simulink model "sim_final_VSS"  (R2019a)
settings: Solver=FixedStepAuto  StartTime=0.0  StopTime=45  FixedStep=1e-2  RelTol=1e-3  EnableMultiTasking=on
values from neighbouring files (symbols this model uses):
  a = 47    [mod1s.m]
  b = -35    [mod1s.m]
  C1 = 0.76    [mod1s.m]
  C2 = 11    [mod1s.m]
  d = 0.5    [mod1s.m]
  ds = 1    [mod1s.m]
  h = 4    [mod1s.m]
  K = 19    [mod1s.m]
  k1 = 3    [mod1s.m]
  k2 = 40    [mod1s.m]
  T = 29    [mod1s.m]
  x0 = -100    [mod1s.m]
  y0 = 0    [mod1s.m]
  z0 = 0    [mod1s.m]
libraries: simulink_extras x1
settings Model: Creator=user  LastModifiedBy=ogure
settings SolverCC: SolverResetMethod=Robust
settings DataIOCC: LimitDataPoints=on  SaveFormat=Array  ReturnWorkspaceOutputs=off  OutputSaveName=x,y,z
settings OptimizationCC: LifeSpan=inf
settings DebuggingCC: SolverPrmCheckMsg=warning  SFUnexpectedBacktrackingDiag=warning  SFNoUnconditionalDefaultTransitionDiag=warning  SFExecutionAtInitializationDiag=none  ArithmeticOperatorsInVariantConditions=warning
settings HardwareCC: ProdBitPerPointer=32  ProdBitPerSizeT=32  ProdBitPerPtrDiffT=32  ProdLargestAtomicFloat=None  ProdIntDivRoundTo=Undefined  ProdEndianess=Unspecified  ProdWordSize=32  ProdHWDeviceType=32-bit Generic
settings ModelReferenceCC: PropagateSignalLabelsOutOfModel=off
settings SFSimCC: SimUseLocalCustomCode=off
settings RTWCC: RTWUseLocalCustomCode=off
settings CodeAppCC: StateflowObjectComments=on
settings GRTTargetCC: TargetLangStandard=C89/C90 (ANSI)  GeneratePreprocessorConditionals=Disable all
settings ConfigComp: CovMetricSettings=dw  CovHtmlReporting=on  CovSaveCumulativeToWorkspaceVar=on  CovSaveSingleToWorkspaceVar=on  CovExternalEMLEnable=off  CovSFcnEnable=off

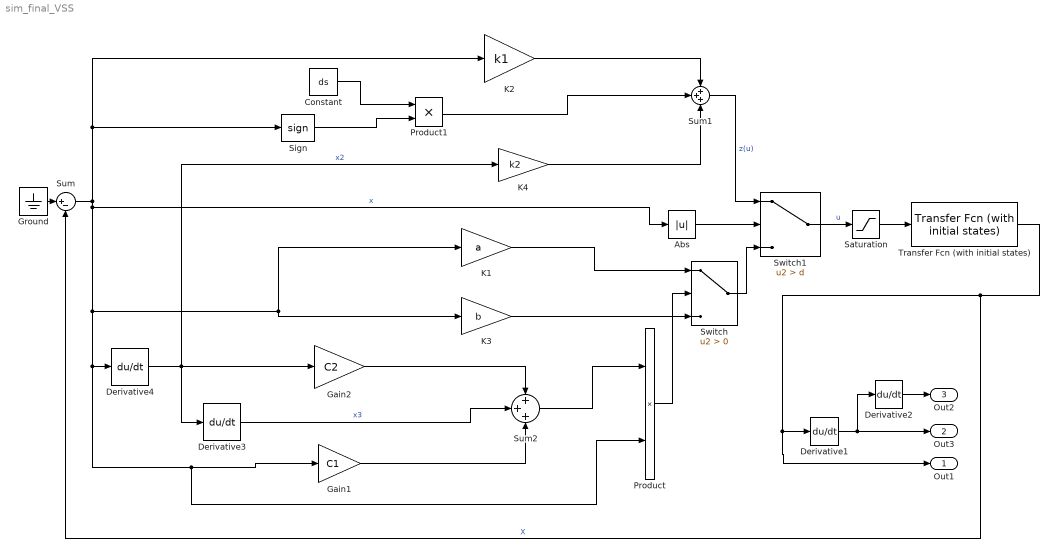
== system sim_final_VSS ==
  Abs : Abs
  Constant : Constant  Value=ds
  Derivative{1..4} (4 alike) : Derivative  CoefficientInTFapproximation=0.00000001
  Gain1 : Gain  Gain=C1
  Gain2 : Gain  Gain=C2
  Ground : Ground
  K1 : Gain  Gain=a
  K2 : Gain  Gain=k1
  K3 : Gain  Gain=b
  K4 : Gain  Gain=k2
  Product : Product
  Product1 : Product
  Saturation : Saturate  UpperLimit=d  LowerLimit=-d
  Sign : Signum
  Sum : Sum  Inputs=|+-
  Sum1 : Sum  Inputs=+++
  Sum2 : Sum  Inputs=+++
  Switch : Switch  Criteria=u2 > Threshold  ZeroCross=off
  Switch1 : Switch  Criteria=u2 > Threshold  Threshold=d  ZeroCross=off
  Transfer Fcn (with initial states) : simulink_extras/Additional Linear/Transfer Fcn (with initial states)  N=K  D=[T^2 2*h*T 1 0]  X0=[z0 y0 x0]
  Out1 : Outport  SignalName=X
  Out3 : Outport  Port=2  SignalName=y
  Out2 : Outport  Port=3  SignalName=z
  wires:
  Transfer Fcn (with initial states)/1 -> Out1/1, Derivative1/1, Sum/2  "X"
  Derivative1/1 -> Derivative2/1, Out3/1
  Derivative2/1 -> Out2/1
  Derivative3/1 -> Sum2/2  "x3"
  Gain1/1 -> Sum2/3
  Sum2/1 -> Product/1
  K1/1 -> Switch/1
  Sum/1 -> Abs/1, K1/1, K3/1, Gain1/1, Product/2, Derivative4/1, K2/1, Sign/1  "x"
  Derivative4/1 -> K4/1, Gain2/1, Derivative3/1  "x2"
  Product/1 -> Switch/2
  Gain2/1 -> Sum2/1
  K3/1 -> Switch/3
  Switch/1 -> Switch1/3
  Sign/1 -> Product1/2
  Constant/1 -> Product1/1
  K2/1 -> Sum1/1
  K4/1 -> Sum1/3
  Product1/1 -> Sum1/2
  Ground/1 -> Sum/1
  Saturation/1 -> Transfer Fcn (with initial states)/1
  Switch1/1 -> Saturation/1  "u"
  Sum1/1 -> Switch1/1  "z(u)"
  Abs/1 -> Switch1/2
